simulink model "SF107A_MotRplCoggCmd"  (R2013b)
settings: Solver=FixedStepDiscrete  SolverMode=SingleTasking  StartTime=0.0  StopTime=1  FixedStep=0.002  RelTol=1e-3
values from neighbouring files (symbols this model uses):
  ARCHGLBPRM_2PI_ULS_F32 = DataDict.Constant    [SF107A_MotRplCoggCmd_DataDict.m]
  ARCHGLBPRM_FLOATZEROTHD_ULS_F32 = DataDict.Constant    [SF107A_MotRplCoggCmd_DataDict.m]
  ININITRNIDXCON_CNT_U16 = DataDict.Constant    [SF107A_MotRplCoggCmd_DataDict.m]
  ITRNIDXCON_CNT_U08 = DataDict.Constant    [SF107A_MotRplCoggCmd_DataDict.m]
  MotRplCoggCmdHrmncOrder1Elec = DataDict.Calibration    [SF107A_MotRplCoggCmd_DataDict.m]
  MotRplCoggCmdHrmncOrder2Elec = DataDict.Calibration    [SF107A_MotRplCoggCmd_DataDict.m]
  MotRplCoggCmdHrmncOrder3Elec = DataDict.Calibration    [SF107A_MotRplCoggCmd_DataDict.m]
  ONEOVER12_MOTREV_F32 = DataDict.Constant    [SF107A_MotRplCoggCmd_DataDict.m]
  ONEOVER2_ULS_F32 = DataDict.Constant    [SF107A_MotRplCoggCmd_DataDict.m]
  ONEOVER2PI_ULS_F32 = DataDict.Constant    [SF107A_MotRplCoggCmd_DataDict.m]
  ONEOVER4_ULS_F32 = DataDict.Constant    [SF107A_MotRplCoggCmd_DataDict.m]
  SINCNVNCON1_ULS_F32 = DataDict.Constant    [SF107A_MotRplCoggCmd_DataDict.m]
  SINCNVNCON2_ULS_F32 = DataDict.Constant    [SF107A_MotRplCoggCmd_DataDict.m]
  SINCNVNCONTBL_ULS_U16 = DataDict.Constant    [SF107A_MotRplCoggCmd_DataDict.m]
undefined symbols (not defined in the file or in its folder): NvmGetErrSts1
libraries: FloatToFixd x8, FixdToFloat x8, NxtrNvM x3, NxtrLim x3, simulink x2, NxtrAbslt x1
(part 3 of 3)

== system SF107A_MotRplCoggCmd/MotRplCoggCmd/MotRplCoggCmdPer1/Regular Calculation/TqRpl Computation/Sine Lookup for Order 1 Phase/Convert to 0 to Pi//2/If Action Subsystem3 ==
  In1 : Inport
  Action Port : ActionPort  ActionType=then
  Add : Sum  Inputs=+-
  Constant1 : Constant  Value=ONEOVER2_ULS_F32
  CopyRight2 : Subsystem  Description=|  mask(Copyright Information){none=on}
      | Copyright info block.                                               
      |                                                                     
      | Place copyright information at the top of every subsystem in design.
      mask prompts: none "No parameters"
      mask help: Place copyright information at the top of every subsystem in design.
      mask Display:
      | NxtrConf = 'Nexteer Confidential';
      | 
      | sys = bdroot; %handle for the current model ("system")
      | first = get_param(sys,'Created');
      | if(isempty(first))
      |     first = datestr(now,'yyyy');
      | else
      |     first = first(end-3:end);  %year is last four digits
      | end
      | 
      | last = get_param(sys,'LastModifiedDate');
      | if isempty(last)
      |     last = datestr(now,'yyyy');
      | else
      |     last = last(end-3:end);
      | end
      | 
      | if strcmp(first,last)
      |     fprintf('%s -- Copyright %s Nexteer',NxtrConf,first)
      | else
      |     fprintf('%s -- %s%s- %s Nexteer',NxtrConf,char(169),first,last)
      | end
  Out1 : Outport
  wires:
  Add/1 -> Out1/1
  Constant1/1 -> Add/1
  In1/1 -> Add/2

== system SF107A_MotRplCoggCmd/MotRplCoggCmd/MotRplCoggCmdPer1/Regular Calculation/TqRpl Computation/Sine Lookup for Order 1 Phase/Convert to 0 to Pi//2/If Action Subsystem4 ==
  Action Port : ActionPort  ActionType=else
  Constant3 : Constant  Value=0  OutDataTypeStr=single
      settings: AttributesFormatString=%<OutDataTypeStr>
  CopyRight2 : Subsystem  Description=|  mask(Copyright Information){none=on}
      | Copyright info block.                                               
      |                                                                     
      | Place copyright information at the top of every subsystem in design.
      mask prompts: none "No parameters"
      mask help: Place copyright information at the top of every subsystem in design.
      mask Display:
      | NxtrConf = 'Nexteer Confidential';
      | 
      | sys = bdroot; %handle for the current model ("system")
      | first = get_param(sys,'Created');
      | if(isempty(first))
      |     first = datestr(now,'yyyy');
      | else
      |     first = first(end-3:end);  %year is last four digits
      | end
      | 
      | last = get_param(sys,'LastModifiedDate');
      | if isempty(last)
      |     last = datestr(now,'yyyy');
      | else
      |     last = last(end-3:end);
      | end
      | 
      | if strcmp(first,last)
      |     fprintf('%s -- Copyright %s Nexteer',NxtrConf,first)
      | else
      |     fprintf('%s -- %s%s- %s Nexteer',NxtrConf,char(169),first,last)
      | end
  Out1 : Outport
  wires:
  Constant3/1 -> Out1/1

== system SF107A_MotRplCoggCmd/MotRplCoggCmd/MotRplCoggCmdPer1/Regular Calculation/TqRpl Computation/Sine Lookup for Order 1 Phase/Convert to 0 to Pi//2/If Action Subsystem8 ==
  In1 : Inport
  Action Port : ActionPort  ActionType=else
  CopyRight2 : Subsystem  Description=|  mask(Copyright Information){none=on}
      | Copyright info block.                                               
      |                                                                     
      | Place copyright information at the top of every subsystem in design.
      mask prompts: none "No parameters"
      mask help: Place copyright information at the top of every subsystem in design.
      mask Display:
      | NxtrConf = 'Nexteer Confidential';
      | 
      | sys = bdroot; %handle for the current model ("system")
      | first = get_param(sys,'Created');
      | if(isempty(first))
      |     first = datestr(now,'yyyy');
      | else
      |     first = first(end-3:end);  %year is last four digits
      | end
      | 
      | last = get_param(sys,'LastModifiedDate');
      | if isempty(last)
      |     last = datestr(now,'yyyy');
      | else
      |     last = last(end-3:end);
      | end
      | 
      | if strcmp(first,last)
      |     fprintf('%s -- Copyright %s Nexteer',NxtrConf,first)
      | else
      |     fprintf('%s -- %s%s- %s Nexteer',NxtrConf,char(169),first,last)
      | end
  Out1 : Outport
  wires:
  In1/1 -> Out1/1

== system SF107A_MotRplCoggCmd/MotRplCoggCmd/MotRplCoggCmdPer1/Regular Calculation/TqRpl Computation/Sine Lookup for Order 2 Phase/Convert to 0 to Pi//2/CopyRight2 ==

== system SF107A_MotRplCoggCmd/MotRplCoggCmd/MotRplCoggCmdPer1/Regular Calculation/TqRpl Computation/Sine Lookup for Order 2 Phase/Convert to 0 to Pi//2/If Action Subsystem ==
  Action Port : ActionPort  ActionType=then
  Constant3 : Constant  OutDataTypeStr=single
      settings: AttributesFormatString=%<OutDataTypeStr>
  CopyRight2 : Subsystem  Description=|  mask(Copyright Information){none=on}
      | Copyright info block.                                               
      |                                                                     
      | Place copyright information at the top of every subsystem in design.
      mask prompts: none "No parameters"
      mask help: Place copyright information at the top of every subsystem in design.
      mask Display:
      | NxtrConf = 'Nexteer Confidential';
      | 
      | sys = bdroot; %handle for the current model ("system")
      | first = get_param(sys,'Created');
      | if(isempty(first))
      |     first = datestr(now,'yyyy');
      | else
      |     first = first(end-3:end);  %year is last four digits
      | end
      | 
      | last = get_param(sys,'LastModifiedDate');
      | if isempty(last)
      |     last = datestr(now,'yyyy');
      | else
      |     last = last(end-3:end);
      | end
      | 
      | if strcmp(first,last)
      |     fprintf('%s -- Copyright %s Nexteer',NxtrConf,first)
      | else
      |     fprintf('%s -- %s%s- %s Nexteer',NxtrConf,char(169),first,last)
      | end
  Out1 : Outport
  wires:
  Constant3/1 -> Out1/1

== system SF107A_MotRplCoggCmd/MotRplCoggCmd/MotRplCoggCmdPer1/Regular Calculation/TqRpl Computation/Sine Lookup for Order 2 Phase/Convert to 0 to Pi//2/If Action Subsystem1 ==
  Action Port : ActionPort  ActionType=then
  Constant1 : Constant  OutDataTypeStr=single
      settings: AttributesFormatString=%<OutDataTypeStr>
  Constant2 : Constant  Value=ONEOVER2_ULS_F32
  CopyRight2 : Subsystem  Description=|  mask(Copyright Information){none=on}
      | Copyright info block.                                               
      |                                                                     
      | Place copyright information at the top of every subsystem in design.
      mask prompts: none "No parameters"
      mask help: Place copyright information at the top of every subsystem in design.
      mask Display:
      | NxtrConf = 'Nexteer Confidential';
      | 
      | sys = bdroot; %handle for the current model ("system")
      | first = get_param(sys,'Created');
      | if(isempty(first))
      |     first = datestr(now,'yyyy');
      | else
      |     first = first(end-3:end);  %year is last four digits
      | end
      | 
      | last = get_param(sys,'LastModifiedDate');
      | if isempty(last)
      |     last = datestr(now,'yyyy');
      | else
      |     last = last(end-3:end);
      | end
      | 
      | if strcmp(first,last)
      |     fprintf('%s -- Copyright %s Nexteer',NxtrConf,first)
      | else
      |     fprintf('%s -- %s%s- %s Nexteer',NxtrConf,char(169),first,last)
      | end
  Unary Minus : UnaryMinus
  Unary Minus1 : UnaryMinus
  Out1 : Outport
  Sign : Outport  Port=2
  wires:
  Constant1/1 -> Unary Minus1/1
  Constant2/1 -> Unary Minus/1
  Unary Minus/1 -> Out1/1
  Unary Minus1/1 -> Sign/1

== system SF107A_MotRplCoggCmd/MotRplCoggCmd/MotRplCoggCmdPer1/Regular Calculation/TqRpl Computation/Sine Lookup for Order 2 Phase/Convert to 0 to Pi//2/If Action Subsystem2 ==
  Action Port : ActionPort  ActionType=else
  Constant1 : Constant  OutDataTypeStr=single
      settings: AttributesFormatString=%<OutDataTypeStr>
  Constant2 : Constant  Value=0  OutDataTypeStr=single
      settings: AttributesFormatString=%<OutDataTypeStr>
  CopyRight2 : Subsystem  Description=|  mask(Copyright Information){none=on}
      | Copyright info block.                                               
      |                                                                     
      | Place copyright information at the top of every subsystem in design.
      mask prompts: none "No parameters"
      mask help: Place copyright information at the top of every subsystem in design.
      mask Display:
      | NxtrConf = 'Nexteer Confidential';
      | 
      | sys = bdroot; %handle for the current model ("system")
      | first = get_param(sys,'Created');
      | if(isempty(first))
      |     first = datestr(now,'yyyy');
      | else
      |     first = first(end-3:end);  %year is last four digits
      | end
      | 
      | last = get_param(sys,'LastModifiedDate');
      | if isempty(last)
      |     last = datestr(now,'yyyy');
      | else
      |     last = last(end-3:end);
      | end
      | 
      | if strcmp(first,last)
      |     fprintf('%s -- Copyright %s Nexteer',NxtrConf,first)
      | else
      |     fprintf('%s -- %s%s- %s Nexteer',NxtrConf,char(169),first,last)
      | end
  Out1 : Outport
  Sign : Outport  Port=2
  wires:
  Constant2/1 -> Out1/1
  Constant1/1 -> Sign/1

== system SF107A_MotRplCoggCmd/MotRplCoggCmd/MotRplCoggCmdPer1/Regular Calculation/TqRpl Computation/Sine Lookup for Order 2 Phase/Convert to 0 to Pi//2/If Action Subsystem3 ==
  In1 : Inport
  Action Port : ActionPort  ActionType=then
  Add : Sum  Inputs=+-
  Constant1 : Constant  Value=ONEOVER2_ULS_F32
  CopyRight2 : Subsystem  Description=|  mask(Copyright Information){none=on}
      | Copyright info block.                                               
      |                                                                     
      | Place copyright information at the top of every subsystem in design.
      mask prompts: none "No parameters"
      mask help: Place copyright information at the top of every subsystem in design.
      mask Display:
      | NxtrConf = 'Nexteer Confidential';
      | 
      | sys = bdroot; %handle for the current model ("system")
      | first = get_param(sys,'Created');
      | if(isempty(first))
      |     first = datestr(now,'yyyy');
      | else
      |     first = first(end-3:end);  %year is last four digits
      | end
      | 
      | last = get_param(sys,'LastModifiedDate');
      | if isempty(last)
      |     last = datestr(now,'yyyy');
      | else
      |     last = last(end-3:end);
      | end
      | 
      | if strcmp(first,last)
      |     fprintf('%s -- Copyright %s Nexteer',NxtrConf,first)
      | else
      |     fprintf('%s -- %s%s- %s Nexteer',NxtrConf,char(169),first,last)
      | end
  Out1 : Outport
  wires:
  Add/1 -> Out1/1
  Constant1/1 -> Add/1
  In1/1 -> Add/2

== system SF107A_MotRplCoggCmd/MotRplCoggCmd/MotRplCoggCmdPer1/Regular Calculation/TqRpl Computation/Sine Lookup for Order 2 Phase/Convert to 0 to Pi//2/If Action Subsystem4 ==
  Action Port : ActionPort  ActionType=else
  Constant3 : Constant  Value=0  OutDataTypeStr=single
      settings: AttributesFormatString=%<OutDataTypeStr>
  CopyRight2 : Subsystem  Description=|  mask(Copyright Information){none=on}
      | Copyright info block.                                               
      |                                                                     
      | Place copyright information at the top of every subsystem in design.
      mask prompts: none "No parameters"
      mask help: Place copyright information at the top of every subsystem in design.
      mask Display:
      | NxtrConf = 'Nexteer Confidential';
      | 
      | sys = bdroot; %handle for the current model ("system")
      | first = get_param(sys,'Created');
      | if(isempty(first))
      |     first = datestr(now,'yyyy');
      | else
      |     first = first(end-3:end);  %year is last four digits
      | end
      | 
      | last = get_param(sys,'LastModifiedDate');
      | if isempty(last)
      |     last = datestr(now,'yyyy');
      | else
      |     last = last(end-3:end);
      | end
      | 
      | if strcmp(first,last)
      |     fprintf('%s -- Copyright %s Nexteer',NxtrConf,first)
      | else
      |     fprintf('%s -- %s%s- %s Nexteer',NxtrConf,char(169),first,last)
      | end
  Out1 : Outport
  wires:
  Constant3/1 -> Out1/1

== system SF107A_MotRplCoggCmd/MotRplCoggCmd/MotRplCoggCmdPer1/Regular Calculation/TqRpl Computation/Sine Lookup for Order 2 Phase/Convert to 0 to Pi//2/If Action Subsystem8 ==
  In1 : Inport
  Action Port : ActionPort  ActionType=else
  CopyRight2 : Subsystem  Description=|  mask(Copyright Information){none=on}
      | Copyright info block.                                               
      |                                                                     
      | Place copyright information at the top of every subsystem in design.
      mask prompts: none "No parameters"
      mask help: Place copyright information at the top of every subsystem in design.
      mask Display:
      | NxtrConf = 'Nexteer Confidential';
      | 
      | sys = bdroot; %handle for the current model ("system")
      | first = get_param(sys,'Created');
      | if(isempty(first))
      |     first = datestr(now,'yyyy');
      | else
      |     first = first(end-3:end);  %year is last four digits
      | end
      | 
      | last = get_param(sys,'LastModifiedDate');
      | if isempty(last)
      |     last = datestr(now,'yyyy');
      | else
      |     last = last(end-3:end);
      | end
      | 
      | if strcmp(first,last)
      |     fprintf('%s -- Copyright %s Nexteer',NxtrConf,first)
      | else
      |     fprintf('%s -- %s%s- %s Nexteer',NxtrConf,char(169),first,last)
      | end
  Out1 : Outport
  wires:
  In1/1 -> Out1/1

== system SF107A_MotRplCoggCmd/MotRplCoggCmd/MotRplCoggCmdPer1/Regular Calculation/TqRpl Computation/Sine Lookup for Order 3 Phase/Convert to 0 to Pi//2/CopyRight2 ==

== system SF107A_MotRplCoggCmd/MotRplCoggCmd/MotRplCoggCmdPer1/Regular Calculation/TqRpl Computation/Sine Lookup for Order 3 Phase/Convert to 0 to Pi//2/If Action Subsystem ==
  Action Port : ActionPort  ActionType=then
  Constant3 : Constant  OutDataTypeStr=single
      settings: AttributesFormatString=%<OutDataTypeStr>
  CopyRight2 : Subsystem  Description=|  mask(Copyright Information){none=on}
      | Copyright info block.                                               
      |                                                                     
      | Place copyright information at the top of every subsystem in design.
      mask prompts: none "No parameters"
      mask help: Place copyright information at the top of every subsystem in design.
      mask Display:
      | NxtrConf = 'Nexteer Confidential';
      | 
      | sys = bdroot; %handle for the current model ("system")
      | first = get_param(sys,'Created');
      | if(isempty(first))
      |     first = datestr(now,'yyyy');
      | else
      |     first = first(end-3:end);  %year is last four digits
      | end
      | 
      | last = get_param(sys,'LastModifiedDate');
      | if isempty(last)
      |     last = datestr(now,'yyyy');
      | else
      |     last = last(end-3:end);
      | end
      | 
      | if strcmp(first,last)
      |     fprintf('%s -- Copyright %s Nexteer',NxtrConf,first)
      | else
      |     fprintf('%s -- %s%s- %s Nexteer',NxtrConf,char(169),first,last)
      | end
  Out1 : Outport
  wires:
  Constant3/1 -> Out1/1

== system SF107A_MotRplCoggCmd/MotRplCoggCmd/MotRplCoggCmdPer1/Regular Calculation/TqRpl Computation/Sine Lookup for Order 3 Phase/Convert to 0 to Pi//2/If Action Subsystem1 ==
  Action Port : ActionPort  ActionType=then
  Constant1 : Constant  OutDataTypeStr=single
      settings: AttributesFormatString=%<OutDataTypeStr>
  Constant2 : Constant  Value=ONEOVER2_ULS_F32
  CopyRight2 : Subsystem  Description=|  mask(Copyright Information){none=on}
      | Copyright info block.                                               
      |                                                                     
      | Place copyright information at the top of every subsystem in design.
      mask prompts: none "No parameters"
      mask help: Place copyright information at the top of every subsystem in design.
      mask Display:
      | NxtrConf = 'Nexteer Confidential';
      | 
      | sys = bdroot; %handle for the current model ("system")
      | first = get_param(sys,'Created');
      | if(isempty(first))
      |     first = datestr(now,'yyyy');
      | else
      |     first = first(end-3:end);  %year is last four digits
      | end
      | 
      | last = get_param(sys,'LastModifiedDate');
      | if isempty(last)
      |     last = datestr(now,'yyyy');
      | else
      |     last = last(end-3:end);
      | end
      | 
      | if strcmp(first,last)
      |     fprintf('%s -- Copyright %s Nexteer',NxtrConf,first)
      | else
      |     fprintf('%s -- %s%s- %s Nexteer',NxtrConf,char(169),first,last)
      | end
  Unary Minus : UnaryMinus
  Unary Minus1 : UnaryMinus
  Out1 : Outport
  Sign : Outport  Port=2
  wires:
  Constant1/1 -> Unary Minus1/1
  Constant2/1 -> Unary Minus/1
  Unary Minus/1 -> Out1/1
  Unary Minus1/1 -> Sign/1

== system SF107A_MotRplCoggCmd/MotRplCoggCmd/MotRplCoggCmdPer1/Regular Calculation/TqRpl Computation/Sine Lookup for Order 3 Phase/Convert to 0 to Pi//2/If Action Subsystem2 ==
  Action Port : ActionPort  ActionType=else
  Constant1 : Constant  OutDataTypeStr=single
      settings: AttributesFormatString=%<OutDataTypeStr>
  Constant2 : Constant  Value=0  OutDataTypeStr=single
      settings: AttributesFormatString=%<OutDataTypeStr>
  CopyRight2 : Subsystem  Description=|  mask(Copyright Information){none=on}
      | Copyright info block.                                               
      |                                                                     
      | Place copyright information at the top of every subsystem in design.
      mask prompts: none "No parameters"
      mask help: Place copyright information at the top of every subsystem in design.
      mask Display:
      | NxtrConf = 'Nexteer Confidential';
      | 
      | sys = bdroot; %handle for the current model ("system")
      | first = get_param(sys,'Created');
      | if(isempty(first))
      |     first = datestr(now,'yyyy');
      | else
      |     first = first(end-3:end);  %year is last four digits
      | end
      | 
      | last = get_param(sys,'LastModifiedDate');
      | if isempty(last)
      |     last = datestr(now,'yyyy');
      | else
      |     last = last(end-3:end);
      | end
      | 
      | if strcmp(first,last)
      |     fprintf('%s -- Copyright %s Nexteer',NxtrConf,first)
      | else
      |     fprintf('%s -- %s%s- %s Nexteer',NxtrConf,char(169),first,last)
      | end
  Out1 : Outport
  Sign : Outport  Port=2
  wires:
  Constant2/1 -> Out1/1
  Constant1/1 -> Sign/1

== system SF107A_MotRplCoggCmd/MotRplCoggCmd/MotRplCoggCmdPer1/Regular Calculation/TqRpl Computation/Sine Lookup for Order 3 Phase/Convert to 0 to Pi//2/If Action Subsystem3 ==
  In1 : Inport
  Action Port : ActionPort  ActionType=then
  Add : Sum  Inputs=+-
  Constant1 : Constant  Value=ONEOVER2_ULS_F32
  CopyRight2 : Subsystem  Description=|  mask(Copyright Information){none=on}
      | Copyright info block.                                               
      |                                                                     
      | Place copyright information at the top of every subsystem in design.
      mask prompts: none "No parameters"
      mask help: Place copyright information at the top of every subsystem in design.
      mask Display:
      | NxtrConf = 'Nexteer Confidential';
      | 
      | sys = bdroot; %handle for the current model ("system")
      | first = get_param(sys,'Created');
      | if(isempty(first))
      |     first = datestr(now,'yyyy');
      | else
      |     first = first(end-3:end);  %year is last four digits
      | end
      | 
      | last = get_param(sys,'LastModifiedDate');
      | if isempty(last)
      |     last = datestr(now,'yyyy');
      | else
      |     last = last(end-3:end);
      | end
      | 
      | if strcmp(first,last)
      |     fprintf('%s -- Copyright %s Nexteer',NxtrConf,first)
      | else
      |     fprintf('%s -- %s%s- %s Nexteer',NxtrConf,char(169),first,last)
      | end
  Out1 : Outport
  wires:
  Add/1 -> Out1/1
  Constant1/1 -> Add/1
  In1/1 -> Add/2

== system SF107A_MotRplCoggCmd/MotRplCoggCmd/MotRplCoggCmdPer1/Regular Calculation/TqRpl Computation/Sine Lookup for Order 3 Phase/Convert to 0 to Pi//2/If Action Subsystem4 ==
  Action Port : ActionPort  ActionType=else
  Constant3 : Constant  Value=0  OutDataTypeStr=single
      settings: AttributesFormatString=%<OutDataTypeStr>
  CopyRight2 : Subsystem  Description=|  mask(Copyright Information){none=on}
      | Copyright info block.                                               
      |                                                                     
      | Place copyright information at the top of every subsystem in design.
      mask prompts: none "No parameters"
      mask help: Place copyright information at the top of every subsystem in design.
      mask Display:
      | NxtrConf = 'Nexteer Confidential';
      | 
      | sys = bdroot; %handle for the current model ("system")
      | first = get_param(sys,'Created');
      | if(isempty(first))
      |     first = datestr(now,'yyyy');
      | else
      |     first = first(end-3:end);  %year is last four digits
      | end
      | 
      | last = get_param(sys,'LastModifiedDate');
      | if isempty(last)
      |     last = datestr(now,'yyyy');
      | else
      |     last = last(end-3:end);
      | end
      | 
      | if strcmp(first,last)
      |     fprintf('%s -- Copyright %s Nexteer',NxtrConf,first)
      | else
      |     fprintf('%s -- %s%s- %s Nexteer',NxtrConf,char(169),first,last)
      | end
  Out1 : Outport
  wires:
  Constant3/1 -> Out1/1

== system SF107A_MotRplCoggCmd/MotRplCoggCmd/MotRplCoggCmdPer1/Regular Calculation/TqRpl Computation/Sine Lookup for Order 3 Phase/Convert to 0 to Pi//2/If Action Subsystem8 ==
  In1 : Inport
  Action Port : ActionPort  ActionType=else
  CopyRight2 : Subsystem  Description=|  mask(Copyright Information){none=on}
      | Copyright info block.                                               
      |                                                                     
      | Place copyright information at the top of every subsystem in design.
      mask prompts: none "No parameters"
      mask help: Place copyright information at the top of every subsystem in design.
      mask Display:
      | NxtrConf = 'Nexteer Confidential';
      | 
      | sys = bdroot; %handle for the current model ("system")
      | first = get_param(sys,'Created');
      | if(isempty(first))
      |     first = datestr(now,'yyyy');
      | else
      |     first = first(end-3:end);  %year is last four digits
      | end
      | 
      | last = get_param(sys,'LastModifiedDate');
      | if isempty(last)
      |     last = datestr(now,'yyyy');
      | else
      |     last = last(end-3:end);
      | end
      | 
      | if strcmp(first,last)
      |     fprintf('%s -- Copyright %s Nexteer',NxtrConf,first)
      | else
      |     fprintf('%s -- %s%s- %s Nexteer',NxtrConf,char(169),first,last)
      | end
  Out1 : Outport
  wires:
  In1/1 -> Out1/1

== system SF107A_MotRplCoggCmd/MotRplCoggCmd/MotRplCoggCmdPer1/Regular Calculation/TqRpl Computation/Sine Lookup for Order 1 Phase/Convert to 0 to Pi//2/If Action Subsystem/CopyRight2 ==

== system SF107A_MotRplCoggCmd/MotRplCoggCmd/MotRplCoggCmdPer1/Regular Calculation/TqRpl Computation/Sine Lookup for Order 1 Phase/Convert to 0 to Pi//2/If Action Subsystem1/CopyRight2 ==

== system SF107A_MotRplCoggCmd/MotRplCoggCmd/MotRplCoggCmdPer1/Regular Calculation/TqRpl Computation/Sine Lookup for Order 1 Phase/Convert to 0 to Pi//2/If Action Subsystem2/CopyRight2 ==

== system SF107A_MotRplCoggCmd/MotRplCoggCmd/MotRplCoggCmdPer1/Regular Calculation/TqRpl Computation/Sine Lookup for Order 1 Phase/Convert to 0 to Pi//2/If Action Subsystem3/CopyRight2 ==

== system SF107A_MotRplCoggCmd/MotRplCoggCmd/MotRplCoggCmdPer1/Regular Calculation/TqRpl Computation/Sine Lookup for Order 1 Phase/Convert to 0 to Pi//2/If Action Subsystem4/CopyRight2 ==

== system SF107A_MotRplCoggCmd/MotRplCoggCmd/MotRplCoggCmdPer1/Regular Calculation/TqRpl Computation/Sine Lookup for Order 1 Phase/Convert to 0 to Pi//2/If Action Subsystem8/CopyRight2 ==

== system SF107A_MotRplCoggCmd/MotRplCoggCmd/MotRplCoggCmdPer1/Regular Calculation/TqRpl Computation/Sine Lookup for Order 2 Phase/Convert to 0 to Pi//2/If Action Subsystem/CopyRight2 ==

== system SF107A_MotRplCoggCmd/MotRplCoggCmd/MotRplCoggCmdPer1/Regular Calculation/TqRpl Computation/Sine Lookup for Order 2 Phase/Convert to 0 to Pi//2/If Action Subsystem1/CopyRight2 ==

== system SF107A_MotRplCoggCmd/MotRplCoggCmd/MotRplCoggCmdPer1/Regular Calculation/TqRpl Computation/Sine Lookup for Order 2 Phase/Convert to 0 to Pi//2/If Action Subsystem2/CopyRight2 ==

== system SF107A_MotRplCoggCmd/MotRplCoggCmd/MotRplCoggCmdPer1/Regular Calculation/TqRpl Computation/Sine Lookup for Order 2 Phase/Convert to 0 to Pi//2/If Action Subsystem3/CopyRight2 ==

== system SF107A_MotRplCoggCmd/MotRplCoggCmd/MotRplCoggCmdPer1/Regular Calculation/TqRpl Computation/Sine Lookup for Order 2 Phase/Convert to 0 to Pi//2/If Action Subsystem4/CopyRight2 ==

== system SF107A_MotRplCoggCmd/MotRplCoggCmd/MotRplCoggCmdPer1/Regular Calculation/TqRpl Computation/Sine Lookup for Order 2 Phase/Convert to 0 to Pi//2/If Action Subsystem8/CopyRight2 ==

== system SF107A_MotRplCoggCmd/MotRplCoggCmd/MotRplCoggCmdPer1/Regular Calculation/TqRpl Computation/Sine Lookup for Order 3 Phase/Convert to 0 to Pi//2/If Action Subsystem/CopyRight2 ==

== system SF107A_MotRplCoggCmd/MotRplCoggCmd/MotRplCoggCmdPer1/Regular Calculation/TqRpl Computation/Sine Lookup for Order 3 Phase/Convert to 0 to Pi//2/If Action Subsystem1/CopyRight2 ==

== system SF107A_MotRplCoggCmd/MotRplCoggCmd/MotRplCoggCmdPer1/Regular Calculation/TqRpl Computation/Sine Lookup for Order 3 Phase/Convert to 0 to Pi//2/If Action Subsystem2/CopyRight2 ==

== system SF107A_MotRplCoggCmd/MotRplCoggCmd/MotRplCoggCmdPer1/Regular Calculation/TqRpl Computation/Sine Lookup for Order 3 Phase/Convert to 0 to Pi//2/If Action Subsystem3/CopyRight2 ==

== system SF107A_MotRplCoggCmd/MotRplCoggCmd/MotRplCoggCmdPer1/Regular Calculation/TqRpl Computation/Sine Lookup for Order 3 Phase/Convert to 0 to Pi//2/If Action Subsystem4/CopyRight2 ==

== system SF107A_MotRplCoggCmd/MotRplCoggCmd/MotRplCoggCmdPer1/Regular Calculation/TqRpl Computation/Sine Lookup for Order 3 Phase/Convert to 0 to Pi//2/If Action Subsystem8/CopyRight2 ==
